simulink model "Steering_Subsystem"  (R2018b)
settings: Solver=FixedStepDiscrete  StartTime=0.0  StopTime=20.0  FixedStep=Step_Size  RelTol=1e-3
values from neighbouring files (symbols this model uses):
  Encoder_Counts_Per_Degree = Simulink.Parameter    [init.m]    (also in init_shared_parameters.m)
  Steering_Offset = Simulink.Parameter    [init.m]    (also in init_NXT_Motor.m; init_Steering_Controller.m; init_Steering_Subsystem.m = 45)
libraries: SignalEditorBlockLib x1
settings Model: Creator=tony  LastModifiedBy=tony
settings OptimizationCC: BlockReduction=off
settings DebuggingCC: ConsistencyChecking=error  SignalInfNanChecking=error  SignalRangeChecking=error  AlgebraicLoopMsg=error  SigSpecEnsureSampleTimeMsg=error  IntegerOverflowMsg=error  ParameterUnderflowMsg=error  ParameterPrecisionLossMsg=error  ParameterTunabilityLossMsg=error  SFcnCompatibilityMsg=error  BusObjectLabelMismatch=error  RootOutportRequireBusObject=error  AllowSymbolicDim=off  ModelReferenceVersionMismatchMessage=error  ModelReferenceIOMismatchMessage=error  UnknownTsInhSupMsg=error  StrictBusMsg=ErrorOnBusTreatedAsVector  BusNameAdapt=ErrorWithoutRepair  NonBusSignalsTreatedAsBus=error  SFInvalidInputDataAccessInChartInitDiag=error  SFTransitionOutsideNaturalParentDiag=error  SFUnreachableExecutionPathDiag=error  SFExecutionAtInitializationDiag=error  SFMachineParentedDataDiag=error  IntegerSaturationMsg=error  AllowAutomaticUnitConversions=off
settings SFSimCC: SimUseLocalCustomCode=off  SimParseCustomCode=off

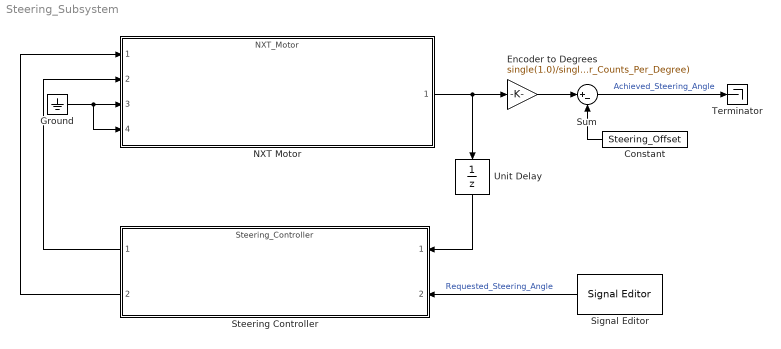
== system Steering_Subsystem ==
  Constant : Constant  Value=Steering_Offset  OutDataTypeStr=single
  Encoder to Degrees : Gain  Gain=single(1.0)/single(Encoder_Counts_Per_Degree)  ParamDataTypeStr=single  OutDataTypeStr=double
  Ground : Ground
  NXT Motor : ModelReference  ModelNameDialog=NXT_Motor  SimulationMode=Normal  ModelReferenceVersion=1.42
  Signal Editor : SignalEditorBlockLib/Signal Editor  FileName=Steering_Requests.mat  ActiveScenario=Scenario  ActiveSignal=SteeringAngle  IsBus=off  OutputBusObjectStr=Bus: BusObject  SampleTime=0  ZeroCross=off  OutputAfterFinalValue=Setting to zero  Unit=inherit
  Steering Controller : ModelReference  ModelNameDialog=Steering_Controller  SimulationMode=Normal  ModelReferenceVersion=1.53
  Sum : Sum  Inputs=|+-
  Terminator : Terminator
  Unit Delay : UnitDelay  InitialCondition=Steering_Offset * single(Encoder_Counts_Per_Degree)  SampleTime=-1
  wires:
  Steering Controller/1 -> NXT Motor/2
  Steering Controller/2 -> NXT Motor/1
  Ground/1 -> NXT Motor/4, NXT Motor/3
  Signal Editor/1 -> Steering Controller/2  "Requested_Steering_Angle"
  NXT Motor/1 -> Encoder to Degrees/1, Unit Delay/1
  Sum/1 -> Terminator/1  "Achieved_Steering_Angle"
  Unit Delay/1 -> Steering Controller/1
  Encoder to Degrees/1 -> Sum/1
  Constant/1 -> Sum/2
